simulink model "lab7_7"  (R2018b)
settings: Solver=FixedStepDiscrete  StartTime=0.0  StopTime=1000000  FixedStep=1  RelTol=1e-3
libraries: hdlsllib x11, simulink x1
settings Model: Creator=mllax8  LastModifiedBy=mllax8

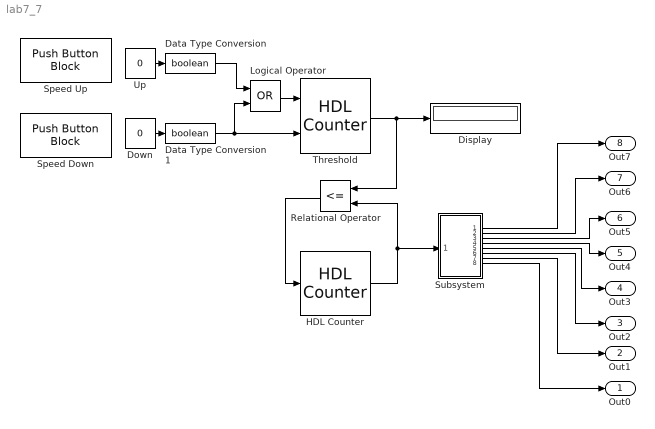
== system lab7_7 ==
  Data Type Conversion : DataTypeConversion  OutDataTypeStr=boolean
  Data Type Conversion1 : DataTypeConversion  OutDataTypeStr=boolean
  Display : Display
  Down : Constant  Value=0
  "HDL Counter " : hdlsllib/Sources/HDL Counter  CountType=Free running  CountInit=0  CountStep=1  CountMax=250000  CountFromType=Initial value  CountFrom=0  CountResetPort=on  CountLoadPort=off  CountEnbPort=off  CountDirPort=off  CountDataType=Unsigned  CountWordLen=18  CountFracLen=0  CountSampTime=1
      settings: SourceProductBaseCode=HD
  Logical Operator : Logic  Operator=OR  AllPortsSameDT=off  OutDataTypeStr=boolean
  Relational Operator : RelationalOperator  Operator=<=  OutDataTypeStr=boolean  RndMeth=Simplest
  Speed Down : PushButtonBlock  WebBlockId=107
  Speed Up : PushButtonBlock  WebBlockId=83
  Subsystem : Subsystem
  Threshold : hdlsllib/Sources/HDL Counter  CountType=Count limited  CountInit=250000  CountStep=1  CountMax=1000000  CountFromType=Initial value  CountFrom=250000  CountResetPort=off  CountLoadPort=off  CountEnbPort=on  CountDirPort=on  CountDataType=Unsigned  CountWordLen=20  CountFracLen=0  CountSampTime=1
      settings: SourceProductBaseCode=HD
  Up : Constant  Value=0
  Out0 : Outport
  Out1 : Outport  Port=2
  Out2 : Outport  Port=3
  Out3 : Outport  Port=4
  Out4 : Outport  Port=5
  Out5 : Outport  Port=6
  Out6 : Outport  Port=7
  Out7 : Outport  Port=8
  wires:
  "HDL Counter "/1 -> Subsystem/1(In1), Relational Operator/2
  Relational Operator/1 -> "HDL Counter "/1
  Subsystem/1(Out1) -> Out7/1
  Subsystem/2(Out2) -> Out6/1
  Subsystem/3(Out3) -> Out5/1
  Subsystem/4(Out4) -> Out4/1
  Subsystem/5(Out5) -> Out3/1
  Subsystem/6(Out6) -> Out2/1
  Subsystem/7(Out7) -> Out1/1
  Subsystem/8(Out8) -> Out0/1
  Threshold/1 -> Display/1, Relational Operator/1
  Logical Operator/1 -> Threshold/1
  Up/1 -> Data Type Conversion/1
  Down/1 -> Data Type Conversion1/1
  Data Type Conversion1/1 -> Threshold/2, Logical Operator/2
  Data Type Conversion/1 -> Logical Operator/1

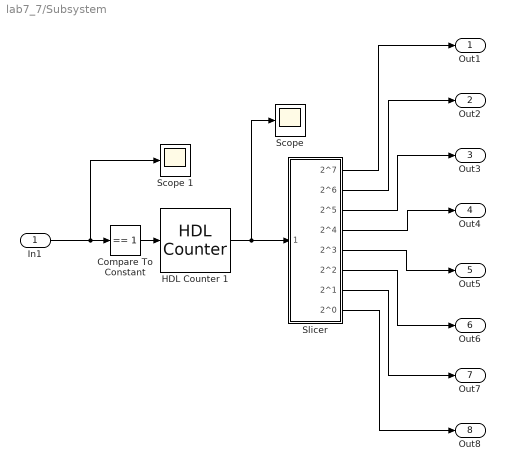
== system lab7_7/Subsystem ==
  In1 : Inport
  Compare To Constant : simulink/Logic and Bit Operations/Compare To Constant  relop===  const=1  OutDataTypeStr=boolean
  HDL Counter 1 : hdlsllib/Sources/HDL Counter  CountType=Free running  CountInit=0  CountStep=1  CountMax=25  CountFromType=Initial value  CountFrom=0  CountResetPort=off  CountLoadPort=off  CountEnbPort=on  CountDirPort=off  CountDataType=Unsigned  CountWordLen=8  CountFracLen=0  CountSampTime=1
      settings: SourceProductBaseCode=HD
  "Scope " : Scope
  Scope 1 : Scope
  Slicer : Subsystem
  Out1 : Outport
  Out2 : Outport  Port=2
  Out3 : Outport  Port=3
  Out4 : Outport  Port=4
  Out5 : Outport  Port=5
  Out6 : Outport  Port=6
  Out7 : Outport  Port=7
  Out8 : Outport  Port=8
  wires:
  Slicer/3(2^5) -> Out3/1
  Slicer/6(2^2) -> Out6/1
  Slicer/4(2^4) -> Out4/1
  Slicer/8("2^0 ") -> Out8/1
  Slicer/2(2^6) -> Out2/1
  HDL Counter 1/1 -> Slicer/1(unsign Int), "Scope "/1
  Slicer/7(2^1) -> Out7/1
  In1/1 -> Scope 1/1, Compare To Constant/1
  Slicer/1(2^7) -> Out1/1
  Slicer/5(2^3) -> Out5/1
  Compare To Constant/1 -> HDL Counter 1/1

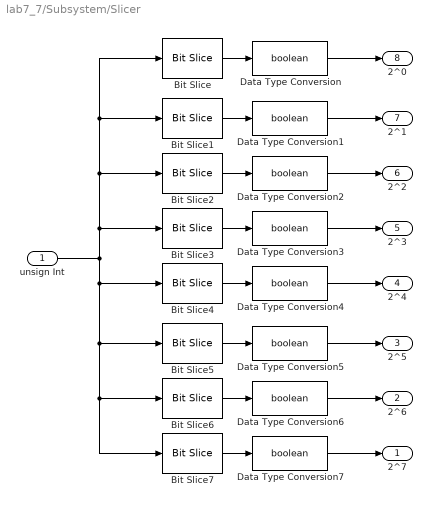
== system lab7_7/Subsystem/Slicer ==
  unsign Int : Inport  OutDataTypeStr=uint8  SampleTime=1
  Bit Slice : hdlsllib/Logic and Bit Operations/Bit Slice  lidx=0  ridx=0
  Bit Slice1 : hdlsllib/Logic and Bit Operations/Bit Slice  lidx=1  ridx=1
  Bit Slice2 : hdlsllib/Logic and Bit Operations/Bit Slice  lidx=2  ridx=2
  Bit Slice3 : hdlsllib/Logic and Bit Operations/Bit Slice  lidx=3  ridx=3
  Bit Slice4 : hdlsllib/Logic and Bit Operations/Bit Slice  lidx=4  ridx=4
  Bit Slice5 : hdlsllib/Logic and Bit Operations/Bit Slice  lidx=5  ridx=5
  Bit Slice6 : hdlsllib/Logic and Bit Operations/Bit Slice  lidx=6  ridx=6
  Bit Slice7 : hdlsllib/Logic and Bit Operations/Bit Slice  lidx=7  ridx=7
  Data Type Conversion{,1..7} (8 alike) : DataTypeConversion  OutDataTypeStr=boolean
  2^7 : Outport
  2^6 : Outport  Port=2
  2^5 : Outport  Port=3
  2^4 : Outport  Port=4
  2^3 : Outport  Port=5
  2^2 : Outport  Port=6
  2^1 : Outport  Port=7
  "2^0 " : Outport  Port=8
  wires:
  Data Type Conversion/1 -> "2^0 "/1
  Data Type Conversion5/1 -> 2^5/1
  Bit Slice1/1 -> Data Type Conversion1/1
  Bit Slice5/1 -> Data Type Conversion5/1
  Bit Slice7/1 -> Data Type Conversion7/1
  Bit Slice2/1 -> Data Type Conversion2/1
  Bit Slice3/1 -> Data Type Conversion3/1
  Data Type Conversion6/1 -> 2^6/1
  Bit Slice4/1 -> Data Type Conversion4/1
  unsign Int/1 -> Bit Slice4/1, Bit Slice5/1, Bit Slice6/1, Bit Slice7/1, Bit Slice3/1, Bit Slice2/1, Bit Slice1/1, Bit Slice/1
  Data Type Conversion1/1 -> 2^1/1
  Data Type Conversion2/1 -> 2^2/1
  Bit Slice/1 -> Data Type Conversion/1
  Bit Slice6/1 -> Data Type Conversion6/1
  Data Type Conversion3/1 -> 2^3/1
  Data Type Conversion4/1 -> 2^4/1
  Data Type Conversion7/1 -> 2^7/1
